simulink model "gm_inc_enc_v26_vnl"  (R2023a)
settings: Solver=FixedStepDiscrete  StartTime=0.0  StopTime=SimulationsDauer  RelTol=1e-3
undefined symbols (not defined in the file or in its folder): CW_CCW_Switch, d_axis_hit_CompareValue, DiscIntNeverNeededParam, f_ISR, IncPerTurn, inital_zero_speed_timeout, n_max, Offset_Position_elec, Offset_Position_mech, OmegaPerOverSampl, Periode, Phase_Delay_A, Phase_Delay_B, PolePair, QuadratureFactor, reciprocal_iterations, T_fpga, T_mech
libraries: simulink x25, hdlmdlgenlib x16, hdlsllib x4, dspsrcs4 x3, dspswit3 x2, spsEdgeDetectorLib x2, simulink_extras x1
(part 3 of 5)

== system gm_inc_enc_v26_vnl/IncEnc_V26_vnl/Check d-Axis-Hit ==
  Count_in : Inport
  IncPerTurn_elek_AXI4 : Inport  Port=2
  Constant : Constant  Value=0  OutDataTypeStr=Inherit: Inherit via back propagation  SampleTime=T_fpga
  Equal : RelationalOperator  Operator===  OutDataTypeStr=boolean  RndMeth=Simplest  InputSameDT=off
  Equal1 : RelationalOperator  Operator===  OutDataTypeStr=boolean  RndMeth=Simplest  InputSameDT=off
  OR : Logic  Operator=OR  AllPortsSameDT=off  OutDataTypeStr=boolean
  d-axis-hit : Outport  VectorParamsAs1DForOutWhenUnconnected=off
  wires:
  OR/1 -> d-axis-hit/1
  Equal1/1 -> OR/2
  Equal/1 -> OR/1
  IncPerTurn_elek_AXI4/1 -> Equal1/2
  Constant/1 -> Equal/2
  Count_in/1 -> Equal/1, Equal1/1

== system gm_inc_enc_v26_vnl/IncEnc_V26_vnl/Check d-Axis-Hit_WithCompare ==
  Count_in : Inport
  Counter_Compare : Inport  Port=2
  Equal : RelationalOperator  Operator===  OutDataTypeStr=boolean  RndMeth=Simplest  InputSameDT=off
  d-axis-hit : Outport  VectorParamsAs1DForOutWhenUnconnected=off
  wires:
  Equal/1 -> d-axis-hit/1
  Count_in/1 -> Equal/1
  Counter_Compare/1 -> Equal/2

== system gm_inc_enc_v26_vnl/IncEnc_V26_vnl/Counter ==
  note: Reset
  note: 1 for one cycle if edge recognized
  Enable_ctr : Inport
  I_line : Inport  Port=2
  Detec_edge : Sum  Inputs=+-  AccumDataTypeStr=int8  OutDataTypeStr=int8
  Reset_flag : Sum  Inputs=+-  AccumDataTypeStr=uint8  OutDataTypeStr=uint8
  reset_old : Delay  DelayLength=1
  reset_old1 : Delay  DelayLength=1
  reset_old_switch : Switch  Criteria=u2 ~= 0  SaturateOnIntegerOverflow=off  InputSameDT=off
  reset_old_switch1 : Switch  Criteria=u2 ~= 0  SaturateOnIntegerOverflow=off  InputSameDT=off
  Edge : Outport  VectorParamsAs1DForOutWhenUnconnected=off
  Reset : Outport  Port=2  VectorParamsAs1DForOutWhenUnconnected=off
  wires:
  Detec_edge/1 -> Edge/1, reset_old_switch1/2  "1 for one cycle if edge recognized"
  reset_old1/1 -> Detec_edge/2, reset_old_switch1/3
  reset_old_switch1/1 -> reset_old1/1
  Enable_ctr/1 -> reset_old_switch1/1, Detec_edge/1
  Reset_flag/1 -> reset_old_switch/2, Reset/1
  reset_old/1 -> Reset_flag/2, reset_old_switch/3
  reset_old_switch/1 -> reset_old/1
  I_line/1 -> reset_old_switch/1, Reset_flag/1

== system gm_inc_enc_v26_vnl/IncEnc_V26_vnl/Counter_Theta_el_wOffset ==
  note: Check if count is to small
  note: Count
  note: Check if count is to big 0-Increments
  Edge : Inport
  Reset : Inport  Port=2
  IncsPerTurn : Inport  Port=3
  Dir : Inport  Port=4
  Position_offset : Inport  Port=5
  Add1 : Sum  AccumDataTypeStr=int16  OutDataTypeStr=int16
  Constant1 : Constant  Value=0  OutDataTypeStr=int16  SampleTime=-1
  Constant2 : Constant  OutDataTypeStr=int16  SampleTime=-1
  Constant3 : Constant  Value=0  OutDataTypeStr=int16  SampleTime=-1
  Constant5 : Constant  Value=-1  OutDataTypeStr=int16  SampleTime=-1
  Relational Operator : RelationalOperator  Operator=>  OutDataTypeStr=boolean  InputSameDT=off
  Relational Operator1 : RelationalOperator  Operator=<=  OutDataTypeStr=boolean  InputSameDT=off
  Resett_switch1 : Switch  Criteria=u2 ~= 0  OutDataTypeStr=uint16  SaturateOnIntegerOverflow=off  InputSameDT=off
  Resett_switch2 : Switch  Criteria=u2 ~= 0  OutDataTypeStr=int16  SaturateOnIntegerOverflow=off  InputSameDT=off
  Resett_switch3 : Switch  Criteria=u2 ~= 0  OutDataTypeStr=int16  SaturateOnIntegerOverflow=off  InputSameDT=off
  Subsystem : Subsystem  Commented=on
  only_use_for_neg_speed : Switch  Threshold=1  SaturateOnIntegerOverflow=off  InputSameDT=off
  reset_old{1..7} (7 alike) : Delay  DelayLength=1
  speed_old_switch1 : Switch  Criteria=u2 ~= 0  SaturateOnIntegerOverflow=off  InputSameDT=off
  speed_old_switch2 : Switch  Threshold=1  SaturateOnIntegerOverflow=off  InputSameDT=off
  count : Outport  VectorParamsAs1DForOutWhenUnconnected=off
  wires:
  speed_old_switch1/1 -> Add1/1
  Constant5/1 -> speed_old_switch2/3
  Relational Operator/1 -> reset_old3/1
  Constant2/1 -> speed_old_switch2/1
  reset_old4/1 -> speed_old_switch1/1
  reset_old5/1 -> Resett_switch3/1, Relational Operator/2
  Resett_switch2/1 -> Resett_switch3/3
  only_use_for_neg_speed/1 -> Resett_switch3/2
  Resett_switch3/1 -> Relational Operator1/1, Resett_switch1/3
  speed_old_switch2/1 -> reset_old4/1
  Relational Operator1/1 -> reset_old2/1
  reset_old3/1 -> Resett_switch1/2
  Resett_switch1/1 -> Relational Operator/1, count/1, reset_old1/1
  Constant1/1 -> only_use_for_neg_speed/1, Relational Operator1/2, Resett_switch1/1
  Constant3/1 -> speed_old_switch1/3
  IncsPerTurn/1 -> reset_old5/1
  Reset/1 -> Resett_switch2/2
  reset_old2/1 -> only_use_for_neg_speed/3
  Edge/1 -> speed_old_switch1/2
  reset_old1/1 -> Add1/2
  Position_offset/1 -> reset_old7/1
  Add1/1 -> Resett_switch2/3
  Dir/1 -> reset_old6/1
  reset_old6/1 -> only_use_for_neg_speed/2, speed_old_switch2/2
  reset_old7/1 -> Resett_switch2/1

== system gm_inc_enc_v26_vnl/IncEnc_V26_vnl/Counter_position ==
  note: Check if count is to small
  note: Check if count is to big 0-Increments
  note: Count
  Edge : Inport
  Reset : Inport  Port=2
  IncsPerTurn : Inport  Port=3
  Dir : Inport  Port=4
  Add1 : Sum  AccumDataTypeStr=int16  OutDataTypeStr=int16
  Constant1 : Constant  Value=0  OutDataTypeStr=int16  SampleTime=-1
  Constant2 : Constant  OutDataTypeStr=int16  SampleTime=-1
  Constant3 : Constant  Value=0  OutDataTypeStr=int16  SampleTime=-1
  Constant4 : Constant  Value=0  OutDataTypeStr=int16  SampleTime=-1
  Constant5 : Constant  Value=-1  OutDataTypeStr=int16  SampleTime=-1
  Relational Operator : RelationalOperator  Operator=>  OutDataTypeStr=boolean  InputSameDT=off
  Relational Operator1 : RelationalOperator  Operator=<=  OutDataTypeStr=boolean  InputSameDT=off
  Resett_switch1 : Switch  Criteria=u2 ~= 0  OutDataTypeStr=uint16  SaturateOnIntegerOverflow=off  InputSameDT=off
  Resett_switch2 : Switch  Criteria=u2 ~= 0  OutDataTypeStr=int16  SaturateOnIntegerOverflow=off  InputSameDT=off
  Resett_switch3 : Switch  Criteria=u2 ~= 0  OutDataTypeStr=int16  SaturateOnIntegerOverflow=off  InputSameDT=off
  only_use_for_neg_speed : Switch  Threshold=1  SaturateOnIntegerOverflow=off  InputSameDT=off
  reset_old{1..6} (6 alike) : Delay  DelayLength=1
  speed_old_switch1 : Switch  Criteria=u2 ~= 0  SaturateOnIntegerOverflow=off  InputSameDT=off
  speed_old_switch2 : Switch  Threshold=1  SaturateOnIntegerOverflow=off  InputSameDT=off
  count : Outport  VectorParamsAs1DForOutWhenUnconnected=off
  wires:
  Constant1/1 -> Resett_switch2/1
  reset_old1/1 -> Add1/2
  reset_old5/1 -> Resett_switch3/1, Relational Operator/2
  reset_old2/1 -> only_use_for_neg_speed/3
  reset_old3/1 -> Resett_switch1/2
  Resett_switch1/1 -> count/1, reset_old1/1, Relational Operator/1
  reset_old6/1 -> speed_old_switch2/2, only_use_for_neg_speed/2
  IncsPerTurn/1 -> reset_old5/1
  reset_old4/1 -> speed_old_switch1/1
  only_use_for_neg_speed/1 -> Resett_switch3/2
  Relational Operator1/1 -> reset_old2/1
  Resett_switch3/1 -> Resett_switch1/3, Relational Operator1/1
  Resett_switch2/1 -> Resett_switch3/3
  Constant4/1 -> Resett_switch1/1, Relational Operator1/2, only_use_for_neg_speed/1
  Relational Operator/1 -> reset_old3/1
  speed_old_switch2/1 -> reset_old4/1
  Constant5/1 -> speed_old_switch2/3
  Dir/1 -> reset_old6/1
  Constant2/1 -> speed_old_switch2/1
  Constant3/1 -> speed_old_switch1/3
  speed_old_switch1/1 -> Add1/1
  Add1/1 -> Resett_switch2/3
  Edge/1 -> speed_old_switch1/2  "1 for one cycle if edge recognized"
  Reset/1 -> Resett_switch2/2

== system gm_inc_enc_v26_vnl/IncEnc_V26_vnl/Counter_position_wOffset ==
  note: Check if count is to big 0-Increments
  note: Count
  note: Check if count is to small
  Edge : Inport
  Reset : Inport  Port=2
  IncsPerTurn : Inport  Port=3
  Dir : Inport  Port=4
  Position_offset : Inport  Port=5
  Add1 : Sum  AccumDataTypeStr=int16  OutDataTypeStr=int16
  Constant1 : Constant  Value=0  OutDataTypeStr=int16  SampleTime=-1
  Constant2 : Constant  OutDataTypeStr=int16  SampleTime=-1
  Constant3 : Constant  Value=0  OutDataTypeStr=int16  SampleTime=-1
  Constant5 : Constant  Value=-1  OutDataTypeStr=int16  SampleTime=-1
  Relational Operator : RelationalOperator  Operator=>  OutDataTypeStr=boolean  InputSameDT=off
  Relational Operator1 : RelationalOperator  Operator=<=  OutDataTypeStr=boolean  InputSameDT=off
  Resett_switch1 : Switch  Criteria=u2 ~= 0  OutDataTypeStr=uint16  SaturateOnIntegerOverflow=off  InputSameDT=off
  Resett_switch2 : Switch  Criteria=u2 ~= 0  OutDataTypeStr=int16  SaturateOnIntegerOverflow=off  InputSameDT=off
  Resett_switch3 : Switch  Criteria=u2 ~= 0  OutDataTypeStr=int16  SaturateOnIntegerOverflow=off  InputSameDT=off
  Subsystem : Subsystem  Commented=on
  only_use_for_neg_speed : Switch  Threshold=1  SaturateOnIntegerOverflow=off  InputSameDT=off
  reset_old{1..7} (7 alike) : Delay  DelayLength=1
  speed_old_switch1 : Switch  Criteria=u2 ~= 0  SaturateOnIntegerOverflow=off  InputSameDT=off
  speed_old_switch2 : Switch  Threshold=1  SaturateOnIntegerOverflow=off  InputSameDT=off
  count : Outport  VectorParamsAs1DForOutWhenUnconnected=off
  wires:
  reset_old7/1 -> Resett_switch2/1
  reset_old6/1 -> speed_old_switch2/2, only_use_for_neg_speed/2
  Dir/1 -> reset_old6/1
  Add1/1 -> Resett_switch2/3
  Position_offset/1 -> reset_old7/1
  reset_old1/1 -> Add1/2
  Edge/1 -> speed_old_switch1/2
  reset_old2/1 -> only_use_for_neg_speed/3
  Reset/1 -> Resett_switch2/2
  IncsPerTurn/1 -> reset_old5/1
  Constant3/1 -> speed_old_switch1/3
  Constant1/1 -> Resett_switch1/1, Relational Operator1/2, only_use_for_neg_speed/1
  Resett_switch1/1 -> reset_old1/1, count/1, Relational Operator/1
  reset_old3/1 -> Resett_switch1/2
  Relational Operator1/1 -> reset_old2/1
  speed_old_switch2/1 -> reset_old4/1
  Resett_switch3/1 -> Resett_switch1/3, Relational Operator1/1
  only_use_for_neg_speed/1 -> Resett_switch3/2
  Resett_switch2/1 -> Resett_switch3/3
  reset_old5/1 -> Relational Operator/2, Resett_switch3/1
  reset_old4/1 -> speed_old_switch1/1
  Constant2/1 -> speed_old_switch2/1
  Relational Operator/1 -> reset_old3/1
  Constant5/1 -> speed_old_switch2/3
  speed_old_switch1/1 -> Add1/1

== system gm_inc_enc_v26_vnl/IncEnc_V26_vnl/Direction ==
  A : Inport
  B : Inport  Port=2
  Add : Sum  Inputs=+-  AccumDataTypeStr=fixdt(1,4,0)  OutDataTypeStr=fixdt(1,4,0)
  Add1 : Sum  Inputs=+-  AccumDataTypeStr=fixdt(1,4,0)  OutDataTypeStr=fixdt(1,4,0)
  Add2 : Sum  AccumDataTypeStr=fixdt(1,4,0)  OutDataTypeStr=fixdt(1,4,0)
  Change : Sum  AccumDataTypeStr=fixdt(1,4,0)  OutDataTypeStr=fixdt(1,4,0)
  Change1 : Delay  DelayLength=1
  Save_Direction : Switch  Criteria=u2 ~= 0  Threshold=0.1  OutDataTypeStr=fixdt(1,4,0)  SaturateOnIntegerOverflow=off  InputSameDT=off
  T_count_switch : Switch  Threshold=1  OutDataTypeStr=Inherit: Inherit via back propagation  SaturateOnIntegerOverflow=off  InputSameDT=off
  TrnLeft : Sum  Inputs=+-  AccumDataTypeStr=fixdt(1,4,0)  OutDataTypeStr=fixdt(1,4,0)
  TrnRight : Sum  Inputs=+-  AccumDataTypeStr=fixdt(1,4,0)  OutDataTypeStr=fixdt(1,4,0)
  TurnLeft : Constant  Value=-1  OutDataTypeStr=fixdt(1,4,0)  SampleTime=-1
  TurnRight : Constant  OutDataTypeStr=fixdt(1,4,0)  SampleTime=-1
  count_old : Delay  DelayLength=1
  count_old1 : Delay  DelayLength=1
  count_old2 : Delay  DelayLength=1
  count_old_switch : Switch  Criteria=u2 ~= 0  OutDataTypeStr=Inherit: Inherit via back propagation  SaturateOnIntegerOverflow=off  InputSameDT=off
  count_old_switch1 : Switch  Criteria=u2 ~= 0  OutDataTypeStr=Inherit: Inherit via back propagation  SaturateOnIntegerOverflow=off  InputSameDT=off
  new_value : Delay  DelayLength=1
  nothing : Constant  Value=0  OutDataTypeStr=fixdt(1,4,0)  SampleTime=-1
  nothing1 : Constant  Value=0  OutDataTypeStr=fixdt(1,4,0)  SampleTime=-1
  speed_old_switch : Switch  Threshold=1  OutDataTypeStr=Inherit: Inherit via back propagation  SaturateOnIntegerOverflow=off  InputSameDT=off
  Dir : Outport  VectorParamsAs1DForOutWhenUnconnected=off
  wires:
  count_old2/1 -> Dir/1, Save_Direction/3  "Dir"
  Change1/1 -> Save_Direction/2  "Change"
  Change/1 -> Change1/1
  Add2/1 -> new_value/1
  speed_old_switch/1 -> Add2/2, Change/2
  nothing1/1 -> T_count_switch/3
  nothing/1 -> speed_old_switch/3
  TurnLeft/1 -> speed_old_switch/1
  TrnLeft/1 -> speed_old_switch/2  "TrnLeft"
  new_value/1 -> Save_Direction/1
  TrnRight/1 -> T_count_switch/2  "Trn_Right"
  Add1/1 -> count_old_switch1/2, TrnLeft/1  "Edge_B"
  count_old1/1 -> Add1/2, count_old_switch1/3
  count_old_switch1/1 -> count_old1/1
  B/1 -> count_old_switch1/1, Add1/1, TrnRight/2
  Save_Direction/1 -> count_old2/1
  T_count_switch/1 -> Add2/1, Change/1
  Add/1 -> count_old_switch/2, TrnRight/1  "Edge_A"
  TurnRight/1 -> T_count_switch/1
  count_old/1 -> Add/2, count_old_switch/3
  count_old_switch/1 -> count_old/1
  A/1 -> count_old_switch/1, Add/1, TrnLeft/2

== system gm_inc_enc_v26_vnl/IncEnc_V26_vnl/Index_Latch ==
  Reset_in : Inport
  Constant : Constant  OutDataTypeStr=boolean  SampleTime=T_fpga
  Constant4 : Constant  Value=0  OutDataTypeStr=boolean  SampleTime=T_fpga
  Delay : Delay  DelayLength=1
  OR : Logic  Operator=OR  AllPortsSameDT=off  OutDataTypeStr=boolean
  Switch : Switch  Criteria=u2 > Threshold  SaturateOnIntegerOverflow=off  InputSameDT=off
  Index_found : Outport
  wires:
  OR/1 -> Switch/2
  Reset_in/1 -> OR/1
  Switch/1 -> Delay/1, Index_found/1
  Constant/1 -> Switch/1
  Delay/1 -> OR/2
  Constant4/1 -> Switch/3

== system gm_inc_enc_v26_vnl/IncEnc_V26_vnl/count_lines ==
  note: omega by counting lines, can be used for high-speed, but is not recommended for small drives!
      | However, for using this approach, we need a quite long time window in order to get an accurate speed.
      | For small drives a long time window is not acceptable, since the mechanical time constant is small.
      | e.g. using just 100us (since the speed control has this period at 10kHz) we can calculate as following:
      | speed = 5034rpm, Increments = 5000, QuadratureFactor = 4, f_cc = 10000 kHz
      | In the test, 169 lines are counted in 100us in the described example.
      | -> 169*(10000/(4*5000))*60 = 5070rpm (so this is not accurate!)
      | However, a longer time window is not acceptabel for speed control with10kHz. More increments is not common, since 5000 are already a lot!
  note: Count
  note: Check if count is to big in order to safe for value overflow
  note: Set new counter value
  Edge : Inport
  Reset : Inport  Port=2
  IncsPerTurn : Inport  Port=3
  Add1 : Sum  AccumDataTypeStr=int16  OutDataTypeStr=int16
  Constant1 : Constant  Value=0  OutDataTypeStr=int16  SampleTime=-1
  Constant2 : Constant  OutDataTypeStr=int16  SampleTime=-1
  Constant3 : Constant  Value=0  OutDataTypeStr=int16  SampleTime=-1
  Constant4 : Constant  Value=10  OutDataTypeStr=int16  SampleTime=-1
  Relational Operator : RelationalOperator  Operator=>  OutDataTypeStr=boolean  InputSameDT=off
  Reset_when_overflow : Sum  OutDataTypeStr=int16
  Resett_switch1 : Switch  Criteria=u2 ~= 0  OutDataTypeStr=int16  SaturateOnIntegerOverflow=off  InputSameDT=off
  Resett_switch2 : Switch  Criteria=u2 ~= 0  OutDataTypeStr=int16  SaturateOnIntegerOverflow=off  InputSameDT=off
  reset_old{1,3..5} (4 alike) : Delay  DelayLength=1
  reset_old_switch1 : Switch  Criteria=u2 ~= 0  SaturateOnIntegerOverflow=off  InputSameDT=off
  speed_old_switch1 : Switch  Criteria=u2 ~= 0  SaturateOnIntegerOverflow=off  InputSameDT=off
  count : Outport  VectorParamsAs1DForOutWhenUnconnected=off
  wires:
  reset_old_switch1/1 -> count/1, reset_old1/1
  Reset/1 -> Resett_switch2/2, reset_old_switch1/2  "Use new value"
  reset_old1/1 -> reset_old_switch1/3
  reset_old3/1 -> Relational Operator/1, Add1/2, reset_old_switch1/1
  Resett_switch1/1 -> reset_old3/1
  Constant4/1 -> Reset_when_overflow/1
  Constant2/1 -> reset_old4/1
  Add1/1 -> Resett_switch2/3
  IncsPerTurn/1 -> Reset_when_overflow/2
  Constant3/1 -> speed_old_switch1/3
  Constant1/1 -> Resett_switch1/1, Resett_switch2/1
  Edge/1 -> speed_old_switch1/2  "1 for one cycle if edge recognized"
  reset_old4/1 -> speed_old_switch1/1
  Resett_switch2/1 -> Resett_switch1/3
  reset_old5/1 -> Relational Operator/2
  speed_old_switch1/1 -> Add1/1
  Relational Operator/1 -> Resett_switch1/2
  Reset_when_overflow/1 -> reset_old5/1

== system gm_inc_enc_v26_vnl/IncEnc_V26_vnl/digital_filter ==
  A : Inport
  AND : Logic  Inputs=3  IconShape=distinctive  AllPortsSameDT=off  OutDataTypeStr=boolean
  AND1 : Logic  Inputs=3  IconShape=distinctive  AllPortsSameDT=off  OutDataTypeStr=boolean
  Delay1 : Delay  DelayLength=1
  Delay2 : Delay  DelayLength=1
  Delay3 : Delay  DelayLength=1
  NOT : Logic  Operator=NOT  IconShape=distinctive  AllPortsSameDT=off  OutDataTypeStr=boolean
  NOT1 : Logic  Operator=NOT  IconShape=distinctive  AllPortsSameDT=off  OutDataTypeStr=boolean
  NOT2 : Logic  Operator=NOT  IconShape=distinctive  AllPortsSameDT=off  OutDataTypeStr=boolean
  Subsystem1 : Subsystem
  Q : Outport
  wires:
  AND/1 -> Subsystem1/1(S)
  AND1/1 -> Subsystem1/2(R)
  Subsystem1/1(Q) -> Q/1
  Delay1/1 -> Delay2/1, NOT/1, AND/1
  Delay2/1 -> Delay3/1, NOT1/1, AND/2
  Delay3/1 -> NOT2/1, AND/3
  NOT/1 -> AND1/1
  NOT1/1 -> AND1/2
  NOT2/1 -> AND1/3
  A/1 -> Delay1/1

== system gm_inc_enc_v26_vnl/IncEnc_V26_vnl/digital_filter1 ==
  A : Inport
  AND : Logic  Inputs=3  IconShape=distinctive  AllPortsSameDT=off  OutDataTypeStr=boolean
  AND1 : Logic  Inputs=3  IconShape=distinctive  AllPortsSameDT=off  OutDataTypeStr=boolean
  Delay1 : Delay  DelayLength=1
  Delay2 : Delay  DelayLength=1
  Delay3 : Delay  DelayLength=1
  NOT : Logic  Operator=NOT  IconShape=distinctive  AllPortsSameDT=off  OutDataTypeStr=boolean
  NOT1 : Logic  Operator=NOT  IconShape=distinctive  AllPortsSameDT=off  OutDataTypeStr=boolean
  NOT2 : Logic  Operator=NOT  IconShape=distinctive  AllPortsSameDT=off  OutDataTypeStr=boolean
  Subsystem1 : Subsystem
  Q : Outport
  wires:
  A/1 -> Delay1/1
  NOT2/1 -> AND1/3
  NOT1/1 -> AND1/2
  NOT/1 -> AND1/1
  Delay3/1 -> AND/3, NOT2/1
  Delay2/1 -> AND/2, NOT1/1, Delay3/1
  Delay1/1 -> AND/1, NOT/1, Delay2/1
  Subsystem1/1(Q) -> Q/1
  AND1/1 -> Subsystem1/2(R)
  AND/1 -> Subsystem1/1(S)

== system gm_inc_enc_v26_vnl/IncEnc_V26_vnl/digital_filter2 ==
  A : Inport
  AND : Logic  Inputs=3  IconShape=distinctive  AllPortsSameDT=off  OutDataTypeStr=boolean
  AND1 : Logic  Inputs=3  IconShape=distinctive  AllPortsSameDT=off  OutDataTypeStr=boolean
  Delay1 : Delay  DelayLength=1
  Delay2 : Delay  DelayLength=1
  Delay3 : Delay  DelayLength=1
  NOT : Logic  Operator=NOT  IconShape=distinctive  AllPortsSameDT=off  OutDataTypeStr=boolean
  NOT1 : Logic  Operator=NOT  IconShape=distinctive  AllPortsSameDT=off  OutDataTypeStr=boolean
  NOT2 : Logic  Operator=NOT  IconShape=distinctive  AllPortsSameDT=off  OutDataTypeStr=boolean
  Subsystem1 : Subsystem
  Q : Outport
  wires:
  AND/1 -> Subsystem1/1(S)
  AND1/1 -> Subsystem1/2(R)
  Subsystem1/1(Q) -> Q/1
  Delay1/1 -> Delay2/1, NOT/1, AND/1
  Delay2/1 -> Delay3/1, NOT1/1, AND/2
  Delay3/1 -> NOT2/1, AND/3
  NOT/1 -> AND1/1
  NOT1/1 -> AND1/2
  NOT2/1 -> AND1/3
  A/1 -> Delay1/1

== system gm_inc_enc_v26_vnl/IncEnc_V26_vnl/speed1 ==
  A : Inport
  B : Inport  Port=2
  Dir : Inport  Port=3
  OmegaPerOverSampl : Inport  Port=4
  T : Inport  Port=5
  timeout_value : Inport  Port=6  OutDataTypeStr=uint32
  Average : Subsystem
  Delay{1..3,6} (4 alike) : Delay  DelayLength=1  InitialCondition=0
  Demux : Demux
  Logical1 : Logic  Operator=NOT  AllPortsSameDT=off  OutDataTypeStr=boolean
  Logical2 : Logic  Operator=NOT  AllPortsSameDT=off  OutDataTypeStr=boolean
  Mux : Mux
  OR1 : Logic  Operator=OR  Inputs=1  AllPortsSameDT=off  OutDataTypeStr=boolean
  OR2 : Logic  Operator=OR  Inputs=1  AllPortsSameDT=off  OutDataTypeStr=boolean
  OS_factor_logic : Subsystem
      settings: PortSchema="{\"entries\":[{\"content\":{\"sides\":[{\"content\":{\"connectorIds\":[\"In1\",\"In2\",\"In3\",\"In4\",\"Out2\"]},\"type\":\"ConnectorPlacement.EquallySpacedRectSide\",\"uuid\":\"00190a63-1990-4dc8-8561-af6346041cd2\"},{\"content\":{\"connectorIds\":[\"Out1\",\"In5\"],\"side\":\"RIGHT\"},\"type\":\"ConnectorPlacement.EquallySpacedRectSide\",\"uuid\":\"ed8fa1bb-ba76-4f60-9676-d72d7f094a86\"},{\"content\":{\"connectorIds\":[],\"side\":\"TOP\"},\"type\":\"ConnectorPlacement.EquallySpacedRectSide\",\"uuid\":\"16aa4cab-6298-4523-a92b-d078d21511a0\"}]},\"type\":\"ConnectorPlacement.EquallySpacedConnector\",\"uuid\":\"bb0c721d-662f-49b4-b1e3-cc7ff0334cdb\"}],\"packageUris\":[\"http://schema.mathworks.com/mf0/Connector/R2020b\"],\"version\":\"1.0\"}"
  calc_omega : Subsystem  TreatAsAtomicUnit=on
  omega : Outport  VectorParamsAs1DForOutWhenUnconnected=off
  OverSamplFactor : Outport  Port=2
  omega_MA_N4 : Outport  Port=3  VectorParamsAs1DForOutWhenUnconnected=off
  timeout_active : Outport  Port=4  OutDataTypeStr=boolean  VectorParamsAs1DForOutWhenUnconnected=off
  omegaA : Outport  Port=5  VectorParamsAs1DForOutWhenUnconnected=off
  omegaB : Outport  Port=6  VectorParamsAs1DForOutWhenUnconnected=off
  omegaNOTA : Outport  Port=7  VectorParamsAs1DForOutWhenUnconnected=off
  omegaNOTB : Outport  Port=8  VectorParamsAs1DForOutWhenUnconnected=off
  new_measurement : Outport  Port=9  OutDataTypeStr=boolean  VectorParamsAs1DForOutWhenUnconnected=off
  wires:
  Average/1(Omega) -> omega/1
  Delay3/1 -> Mux/4
  Delay2/1 -> Mux/3
  Delay1/1 -> Mux/2
  Delay6/1 -> Mux/1
  OS_factor_logic/1(oversampling_adjusted) -> calc_omega/4(oversampling_state)
  Logical1/1 -> Delay3/1  "NOT_B"
  Logical2/1 -> Delay2/1  "NOT_A"
  calc_omega/4(timeout_active) -> OR1/1
  calc_omega/3(state_count_edges) -> OS_factor_logic/3(state_edges)
  calc_omega/2(NewMeasurement) -> OS_factor_logic/1(new_transisiton), OR2/1  "newMeas"
  calc_omega/1(omega_oversampled) -> Average/1("OmegaIn "), Demux/1  "omega"
  Demux/3 -> omegaNOTA/1
  Demux/4 -> omegaNOTB/1
  Demux/1 -> omegaA/1
  Demux/2 -> omegaB/1
  timeout_value/1 -> calc_omega/5(timeout_value)
  T/1 -> calc_omega/3(T)
  Mux/1 -> calc_omega/1(Encoder Line)
  A/1 -> Delay6/1, Logical2/1  "A"
  Average/2(OmegaOut_MA_N4) -> OS_factor_logic/4(omega), omega_MA_N4/1  "final omega oversampled"
  OR1/1 -> timeout_active/1  "timeout_active_all_ORed"
  OS_factor_logic/2(oversampling_state) -> OverSamplFactor/1  "OS_B"
  OR2/1 -> new_measurement/1, Average/2(NewMeasurement), OS_factor_logic/2(Allow_ToCheckOversampling)  "newMeas_allORed"
  OmegaPerOverSampl/1 -> OS_factor_logic/5(OverSamplOmega)
  B/1 -> Logical1/1, Delay1/1  "B"
  Dir/1 -> calc_omega/2(Dir)

== system gm_inc_enc_v26_vnl/Testfield/Counter_position_wOffset ==
  note: Check if count is to small
  note: Count
  note: Check if count is to big 0-Increments
  Edge : Inport
  Reset : Inport  Port=2
  IncsPerTurn : Inport  Port=3
  Dir : Inport  Port=4
  Position_offset : Inport  Port=5
  Add1 : Sum  AccumDataTypeStr=int16  OutDataTypeStr=int16
  Constant1 : Constant  Value=0  OutDataTypeStr=int16  SampleTime=-1
  Constant2 : Constant  OutDataTypeStr=int16  SampleTime=-1
  Constant3 : Constant  Value=0  OutDataTypeStr=int16  SampleTime=-1
  Constant5 : Constant  Value=-1  OutDataTypeStr=int16  SampleTime=-1
  Relational Operator : RelationalOperator  Operator=>  OutDataTypeStr=boolean  InputSameDT=off
  Relational Operator1 : RelationalOperator  Operator=<=  OutDataTypeStr=boolean  InputSameDT=off
  Resett_switch1 : Switch  Criteria=u2 ~= 0  OutDataTypeStr=uint16  SaturateOnIntegerOverflow=off  InputSameDT=off
  Resett_switch2 : Switch  Criteria=u2 ~= 0  OutDataTypeStr=int16  SaturateOnIntegerOverflow=off  InputSameDT=off
  Resett_switch3 : Switch  Criteria=u2 ~= 0  OutDataTypeStr=int16  SaturateOnIntegerOverflow=off  InputSameDT=off
  Subsystem : Subsystem  Commented=on
  only_use_for_neg_speed : Switch  Threshold=1  SaturateOnIntegerOverflow=off  InputSameDT=off
  reset_old{1..7} (7 alike) : Delay  DelayLength=1
  speed_old_switch1 : Switch  Criteria=u2 ~= 0  SaturateOnIntegerOverflow=off  InputSameDT=off
  speed_old_switch2 : Switch  Threshold=1  SaturateOnIntegerOverflow=off  InputSameDT=off
  count : Outport  VectorParamsAs1DForOutWhenUnconnected=off
  wires:
  speed_old_switch1/1 -> Add1/1
  Constant5/1 -> speed_old_switch2/3
  Relational Operator/1 -> reset_old3/1
  Constant2/1 -> speed_old_switch2/1
  reset_old4/1 -> speed_old_switch1/1
  reset_old5/1 -> Resett_switch3/1, Relational Operator/2
  Resett_switch2/1 -> Resett_switch3/3
  only_use_for_neg_speed/1 -> Resett_switch3/2
  Resett_switch3/1 -> Relational Operator1/1, Resett_switch1/3
  speed_old_switch2/1 -> reset_old4/1
  Relational Operator1/1 -> reset_old2/1
  reset_old3/1 -> Resett_switch1/2
  Resett_switch1/1 -> Relational Operator/1, count/1, reset_old1/1
  Constant1/1 -> only_use_for_neg_speed/1, Relational Operator1/2, Resett_switch1/1
  Constant3/1 -> speed_old_switch1/3
  IncsPerTurn/1 -> reset_old5/1
  Reset/1 -> Resett_switch2/2
  reset_old2/1 -> only_use_for_neg_speed/3
  Edge/1 -> speed_old_switch1/2
  reset_old1/1 -> Add1/2
  Position_offset/1 -> reset_old7/1
  Add1/1 -> Resett_switch2/3
  Dir/1 -> reset_old6/1
  reset_old6/1 -> only_use_for_neg_speed/2, speed_old_switch2/2
  reset_old7/1 -> Resett_switch2/1

== system gm_inc_enc_v26_vnl/Testfield/Index_Latch ==
  Reset_in : Inport
  Constant : Constant  OutDataTypeStr=boolean
  Constant4 : Constant  Value=0  OutDataTypeStr=boolean
  Delay : Delay  DelayLength=1
  OR : Logic  Operator=OR  AllPortsSameDT=off  OutDataTypeStr=boolean
  Switch : Switch  Criteria=u2 > Threshold  SaturateOnIntegerOverflow=off  InputSameDT=off
  Index_found : Outport
  wires:
  Constant4/1 -> Switch/3
  Delay/1 -> OR/2
  Constant/1 -> Switch/1
  Switch/1 -> Index_found/1, Delay/1
  Reset_in/1 -> OR/1
  OR/1 -> Switch/2

== system gm_inc_enc_v26_vnl/Create_Referenz/IncrementalEncoder_Floating/CutTheta_0_2PI ==
  In1 : Inport
  Add7 : Sum  Inputs=+-  OutDataTypeStr=double
  Gain : Gain  Gain=1/(2*pi)
  Gain11 : Gain  Gain=2*pi
  Rounding Function : Rounding
  Out1 : Outport  VectorParamsAs1DForOutWhenUnconnected=off
  wires:
  Gain/1 -> Rounding Function/1
  Rounding Function/1 -> Gain11/1
  Gain11/1 -> Add7/2
  In1/1 -> Gain/1, Add7/1
  Add7/1 -> Out1/1

== system gm_inc_enc_v26_vnl/Create_Referenz/IncrementalEncoder_Floating/n_aus_theta_v4 ==
  theta : Inport
  Abs : Abs  SaturateOnIntegerOverflow=off
  Add : Sum  Inputs=-+
  Add1 : Sum  Inputs=+-
  Gain : Gain  Gain=2*pi
  Gain1 : Gain  Gain=1/T_mech
  Gain2 : Gain  Gain=60/(2*pi)
  Geschwindigkeitsfilter1 : Subsystem
  Rate Limiter2 1/T : RateLimiter  RisingSlewLimit=1/T_mech*10  FallingSlewLimit=-1/T_mech*10  SampleTimeMode=inherited
  Saturation : Saturate  UpperLimit=n_max  LowerLimit=-n_max
  Scope1 : Scope  NumInputPorts=5
  Scope2 : Scope  NumInputPorts=5
  Sign : Signum
  Switch : Switch  Threshold=3  SaturateOnIntegerOverflow=off  InputSameDT=off
  Unit Delay : UnitDelay  SampleTime=-1  HasFrameUpgradeWarning=on
  n : Outport  VectorParamsAs1DForOutWhenUnconnected=off
  wires:
  Switch/1 -> Scope1/3, Gain1/1
  Add/1 -> Scope2/1, Switch/1
  Gain/1 -> Add/1
  Sign/1 -> Gain/1
  Add1/1 -> Scope2/3, Add/2, Abs/1, Scope2/2, Switch/3, Sign/1
  Abs/1 -> Scope1/4, Switch/2
  Gain1/1 -> Scope1/2, Gain2/1
  theta/1 -> Scope2/5, Add1/1, Unit Delay/1
  Unit Delay/1 -> Scope2/4, Add1/2
  Gain2/1 -> Saturation/1
  Geschwindigkeitsfilter1/1(Out1) -> Scope1/5, Rate Limiter2 1/T/1
  Rate Limiter2 1/T/1 -> n/1
  Saturation/1 -> Scope1/1, Geschwindigkeitsfilter1/1(In1)

== system gm_inc_enc_v26_vnl/IncEnc_V26/digital_filter/Subsystem1 ==
  S : Inport  OutDataTypeStr=boolean  PortDimensions=1  SampleTime=1e-08
  R : Inport  Port=2  OutDataTypeStr=boolean  PortDimensions=1  SampleTime=1e-08
  AND : Logic  Operator=NOR  AllPortsSameDT=off  OutDataTypeStr=boolean  SampleTime=1e-08
  AND1 : Logic  Operator=NOR  AllPortsSameDT=off  OutDataTypeStr=boolean  SampleTime=1e-08
  Delay : Delay  DelayLength=double(1)  InitialCondition=0  SampleTime=1e-08
  Q : Outport  SampleTime=1e-08
  wires:
  AND1/1 -> AND/2
  Delay/1 -> AND1/1
  AND/1 -> Delay/1, Q/1
  R/1 -> AND/1
  S/1 -> AND1/2

== system gm_inc_enc_v26_vnl/IncEnc_V26/digital_filter1/Subsystem1 ==
  S : Inport  OutDataTypeStr=boolean  PortDimensions=1  SampleTime=1e-08
  R : Inport  Port=2  OutDataTypeStr=boolean  PortDimensions=1  SampleTime=1e-08
  AND : Logic  Operator=NOR  AllPortsSameDT=off  OutDataTypeStr=boolean  SampleTime=1e-08
  AND1 : Logic  Operator=NOR  AllPortsSameDT=off  OutDataTypeStr=boolean  SampleTime=1e-08
  Delay : Delay  DelayLength=double(1)  InitialCondition=0  SampleTime=1e-08
  Q : Outport  SampleTime=1e-08
  wires:
  AND1/1 -> AND/2
  Delay/1 -> AND1/1
  AND/1 -> Delay/1, Q/1
  R/1 -> AND/1
  S/1 -> AND1/2

== system gm_inc_enc_v26_vnl/IncEnc_V26/digital_filter2/Subsystem1 ==
  S : Inport  OutDataTypeStr=boolean  PortDimensions=1  SampleTime=1e-08
  R : Inport  Port=2  OutDataTypeStr=boolean  PortDimensions=1  SampleTime=1e-08
  AND : Logic  Operator=NOR  AllPortsSameDT=off  OutDataTypeStr=boolean  SampleTime=1e-08
  AND1 : Logic  Operator=NOR  AllPortsSameDT=off  OutDataTypeStr=boolean  SampleTime=1e-08
  Delay : Delay  DelayLength=double(1)  InitialCondition=0  SampleTime=1e-08
  Q : Outport  SampleTime=1e-08
  wires:
  AND1/1 -> AND/2
  Delay/1 -> AND1/1
  AND/1 -> Delay/1, Q/1
  R/1 -> AND/1
  S/1 -> AND1/2

== system gm_inc_enc_v26_vnl/IncEnc_V26/speed1/Average ==
  note: average 4 parallel measurements
  note: moving average of 4 last measurements, which in total results in a moving average of the last 8 samples
  "OmegaIn " : Inport  OutDataTypeStr=fixdt(1, 24, 11)  PortDimensions=[4]  SampleTime=1e-08
  NewMeasurement : Inport  Port=2  OutDataTypeStr=boolean  PortDimensions=1  SampleTime=1e-08
  Delay_Switch : Switch  Criteria=u2 ~= 0  Threshold=double(0)  OutDataTypeStr=fixdt(1, 24, 11)  SampleTime=1e-08  SaturateOnIntegerOverflow=off  InputSameDT=off
  Delay_Switch1 : Switch  Criteria=u2 ~= 0  Threshold=double(0)  OutDataTypeStr=fixdt(1, 24, 11)  SampleTime=1e-08  SaturateOnIntegerOverflow=off  InputSameDT=off
  Delay_Switch2 : Switch  Criteria=u2 ~= 0  Threshold=double(0)  OutDataTypeStr=fixdt(1, 24, 11)  SampleTime=1e-08  SaturateOnIntegerOverflow=off  InputSameDT=off
  Gain : Gain  Gain="fi(0,1,26,26,\"hex\",\"1000000\")"  ParamDataTypeStr=fixdt(1, 26, 26)  OutDataTypeStr=fixdt(1, 24, 11)  SampleTime=1e-08
  Gain1 : Gain  Gain="fi(0,1,26,26,\"hex\",\"1000000\")"  ParamDataTypeStr=fixdt(1, 26, 26)  OutDataTypeStr=fixdt(1, 24, 11)  SampleTime=1e-08
  Sum of Elements{1..2,4..5} (4 alike) : Sum  AccumDataTypeStr=fixdt(1, 25, 11)  OutDataTypeStr=fixdt(1, 25, 11)  SampleTime=1e-08
  Sum of Elements3 : Sum  AccumDataTypeStr=fixdt(1, 26, 11)  OutDataTypeStr=fixdt(1, 26, 11)  SampleTime=1e-08
  Sum of Elements6 : Sum  AccumDataTypeStr=fixdt(1, 26, 11)  OutDataTypeStr=fixdt(1, 26, 11)  SampleTime=1e-08
  rd_{0..8} (9 alike) : Delay  DelayLength=double(1)  InitialCondition=0  SampleTime=1e-08
  t : Demux
  t{1..6} (6 alike) : hdlmdlgenlib/Buffer
  Omega : Outport  SampleTime=1e-08  VectorParamsAs1DForOutWhenUnconnected=off
  OmegaOut_MA_N4 : Outport  Port=2  SampleTime=1e-08  VectorParamsAs1DForOutWhenUnconnected=off
  wires:
  rd_5/1 -> Delay_Switch2/2, Delay_Switch1/2, Delay_Switch/2
  t2/1 -> rd_5/1
  rd_8/1 -> Sum of Elements2/2, Delay_Switch2/3
  t6/1 -> rd_8/1
  rd_7/1 -> Sum of Elements2/1, Delay_Switch2/1, Delay_Switch1/3
  t5/1 -> rd_7/1
  rd_6/1 -> Sum of Elements1/2, Delay_Switch/3, Delay_Switch1/1
  t4/1 -> rd_6/1
  rd_4/1 -> Sum of Elements1/1
  rd_1/1 -> Sum of Elements5/1
  rd_3/1 -> Sum of Elements5/2
  rd_2/1 -> Sum of Elements4/2
  rd_0/1 -> Sum of Elements4/1
  Delay_Switch2/1 -> t6/1
  Delay_Switch1/1 -> t5/1
  Delay_Switch/1 -> t4/1
  NewMeasurement/1 -> t2/1
  "OmegaIn "/1 -> t/1
  t/4 -> rd_3/1
  t/3 -> rd_1/1
  t/2 -> rd_2/1
  t/1 -> rd_0/1
  t3/1 -> rd_4/1
  Sum of Elements6/1 -> Gain1/1
  Sum of Elements5/1 -> Sum of Elements6/2
  Sum of Elements4/1 -> Sum of Elements6/1
  Sum of Elements3/1 -> Gain/1
  Sum of Elements2/1 -> Sum of Elements3/2
  Sum of Elements1/1 -> Sum of Elements3/1
  Gain1/1 -> t1/1
  Gain/1 -> OmegaOut_MA_N4/1
  t1/1 -> Delay_Switch/1, Omega/1, t3/1

== system gm_inc_enc_v26_vnl/IncEnc_V26/speed1/OS_factor_logic ==
  new_transisiton : Inport  OutDataTypeStr=boolean  PortDimensions=[4]  SampleTime=1e-08
  Allow_ToCheckOversampling : Inport  Port=2  OutDataTypeStr=boolean  PortDimensions=1  SampleTime=1e-08
  state_edges : Inport  Port=3  OutDataTypeStr=int16  PortDimensions=[4]  SampleTime=1e-08
  omega : Inport  Port=4  OutDataTypeStr=fixdt(1, 24, 11)  PortDimensions=1  SampleTime=1e-08
  OverSamplOmega : Inport  Port=5  OutDataTypeStr=fixdt(1, 24, 11)  PortDimensions=1  SampleTime=1e-08
  Abs : Abs  SampleTime=1e-08  OutDataTypeStr=fixdt(1, 24, 11)  SaturateOnIntegerOverflow=off
  Data Type Conversion1 : DataTypeConversion  OutDataTypeStr=fixdt(0,16,0)
  Delay7_Initial_Val : Constant  OutDataTypeStr=uint16  SampleTime=1e-08
  Delay7_ctrl_const : Constant  OutDataTypeStr=boolean  SampleTime=1e-08
  Delay7_switch : Switch  Criteria=u2 ~= 0  Threshold=double(0)  OutDataTypeStr=uint16  SampleTime=1e-08  SaturateOnIntegerOverflow=off  InputSameDT=off
  Sum : Sum  Inputs=+-  AccumDataTypeStr=uint16  OutDataTypeStr=uint16  SampleTime=1e-08
  align_oversamples : Subsystem
  oversample_factor : Subsystem
  rd_{0..3} (4 alike) : Delay  DelayLength=double(1)  InitialCondition=0  SampleTime=1e-08
  oversampling_adjusted : Outport  PortDimensions=4  SampleTime=1e-08
  oversampling_state : Outport  Port=2  SampleTime=1e-08
  wires:
  rd_0/1 -> Delay7_switch/2
  rd_1/1 -> oversample_factor/5(InternalOmega)
  rd_2/1 -> Delay7_switch/1
  rd_3/1 -> Sum/2
  Delay7_ctrl_const/1 -> rd_0/1
  Delay7_Initial_Val/1 -> Delay7_switch/3
  oversample_factor/2(InternalOmega_Out) -> rd_1/1
  oversample_factor/1(state_Out) -> rd_2/1
  align_oversamples/1(delay_output) -> rd_3/1
  Sum/1 -> oversampling_adjusted/1
  Delay7_switch/1 -> align_oversamples/1(oversampling_factor), oversample_factor/4(state), Data Type Conversion1/1, Sum/1
  Data Type Conversion1/1 -> oversampling_state/1
  Abs/1 -> oversample_factor/2(ReadBack_Omega)
  OverSamplOmega/1 -> oversample_factor/3(OverSamplOmega)
  omega/1 -> Abs/1
  state_edges/1 -> align_oversamples/3(states)
  Allow_ToCheckOversampling/1 -> oversample_factor/1(AllowCheckOverSampl)
  new_transisiton/1 -> align_oversamples/2(new_transition)

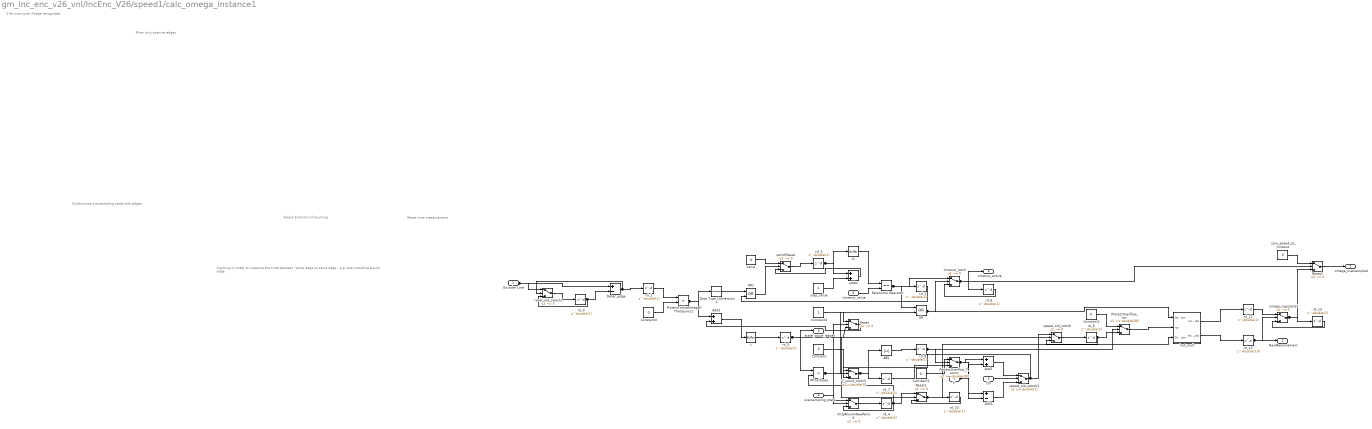
== system gm_inc_enc_v26_vnl/IncEnc_V26/speed1/calc_omega_instance1 ==
  note: Synchronize oversampling state with edges
  note: Filter only positive edges
  note: Select direction of counting
  note: 1 for one cycle if edge recognized
  note: Reset time measurement
  note: Count up in order to measure the time between "same edge to same edge", e.g. every positive A-Line edge
  Encoder Line : Inport  OutDataTypeStr=boolean  PortDimensions=1  SampleTime=1e-08
  Dir : Inport  Port=2  OutDataTypeStr=fixdt(1, 4, 0)  PortDimensions=1  SampleTime=1e-08
  T : Inport  Port=3  OutDataTypeStr=fixdt(1, 38, 32)  PortDimensions=1  SampleTime=1e-08
  oversampling_state : Inport  Port=4  OutDataTypeStr=uint16  PortDimensions=1  SampleTime=1e-08
  timeout_value : Inport  Port=5  OutDataTypeStr=uint32  PortDimensions=1  SampleTime=1e-08
  ABS : Abs  SampleTime=1e-08  OutDataTypeStr=fixdt(1, 38, 32)  SaturateOnIntegerOverflow=off
  Add1 : Sum  AccumDataTypeStr=fixdt(1, 38, 32)  OutDataTypeStr=fixdt(1, 38, 32)  SampleTime=1e-08
  Add2 : Sum  Inputs=+-  AccumDataTypeStr=fixdt(1, 38, 32)  OutDataTypeStr=fixdt(1, 38, 32)  SampleTime=1e-08
  Add3 : Sum  AccumDataTypeStr=int16  OutDataTypeStr=int16  SampleTime=1e-08
  Constant : Constant  Value=0  OutDataTypeStr=fixdt(1, 38, 32)  SampleTime=1e-08
  Constant1 : Constant  Value=0  OutDataTypeStr=fixdt(1, 38, 32)  SampleTime=1e-08
  Constant2 : Constant  Value=0  OutDataTypeStr=fixdt(1, 38, 32)  SampleTime=1e-08
  Constant3 : Constant  Value=0  OutDataTypeStr=int8  SampleTime=1e-08
  Constant4 : Constant  OutDataTypeStr=int8  SampleTime=1e-08
  Data Type Conversion1 : DataTypeConversion  OutDataTypeStr=boolean  SampleTime=1e-08  SaturateOnIntegerOverflow=off  RndMeth=Floor
  Detec_edge : Sum  Inputs=+-  AccumDataTypeStr=int8  OutDataTypeStr=int8  SampleTime=1e-08
  IfFinalState : RelationalOperator  Operator=>  OutDataTypeStr=boolean  SampleTime=1e-08  InputSameDT=off
  OR : Logic  Operator=OR  AllPortsSameDT=off  OutDataTypeStr=boolean  SampleTime=1e-08
  OR1 : Logic  Operator=OR  AllPortsSameDT=off  OutDataTypeStr=boolean  SampleTime=1e-08
  OnlyAllowInNewPeriod : Switch  Criteria=u2 ~= 0  Threshold=double(0)  OutDataTypeStr=uint16  SampleTime=1e-08  SaturateOnIntegerOverflow=off  InputSameDT=off
  ProtectOverflow_T_count : Switch  Threshold=double(30)  OutDataTypeStr=fixdt(1, 38, 32)  SampleTime=1e-08  SaturateOnIntegerOverflow=off  InputSameDT=off
  ProtectOverflow_rps : Switch  Threshold=double(30)  OutDataTypeStr=fixdt(1, 38, 32)  SampleTime=1e-08  SaturateOnIntegerOverflow=off  InputSameDT=off
  ProtectToUseOmegaIfThetaJump1 : RelationalOperator  Operator=>  OutDataTypeStr=fixdt(1,16,0)  SampleTime=1e-08  InputSameDT=off
  Relational Operator : RelationalOperator  Operator===  OutDataTypeStr=boolean  SampleTime=1e-08  InputSameDT=off
  Reset : Switch  Criteria=u2 ~= 0  Threshold=double(0)  OutDataTypeStr=fixdt(1, 24, 11)  SampleTime=1e-08  SaturateOnIntegerOverflow=off  InputSameDT=off
  Reset1 : Switch  Criteria=u2 ~= 0  Threshold=double(0)  OutDataTypeStr=uint16  SampleTime=1e-08  SaturateOnIntegerOverflow=off  InputSameDT=off
  Reset2 : Switch  Criteria=u2 ~= 0  Threshold=double(0)  OutDataTypeStr=fixdt(1, 24, 11)  SampleTime=1e-08  SaturateOnIntegerOverflow=off  InputSameDT=off
  T_count_switch : Switch  Criteria=u2 > Threshold  Threshold=double(0)  OutDataTypeStr=fixdt(1, 38, 32)  SampleTime=1e-08  SaturateOnIntegerOverflow=off  InputSameDT=off
  adder : Sum  AccumDataTypeStr=uint32  OutDataTypeStr=uint32  SampleTime=1e-08
  const : Constant  Value=0  VectorParams1D=off  OutDataTypeStr=uint32  SampleTime=1e-08
  invt_mult : Subsystem
  omega_registered : Switch  Criteria=u2 ~= 0  Threshold=double(0)  OutDataTypeStr=fixdt(1, 24, 11)  SampleTime=1e-08  SaturateOnIntegerOverflow=off  InputSameDT=off
  rd_{0..10,13} (12 alike) : Delay  DelayLength=double(1)  InitialCondition=0  SampleTime=1e-08
  rd_11 : Delay  DelayLength=double(2)  InitialCondition=0  SampleTime=1e-08
  rd_12 : Delay  DelayLength=double(19)  InitialCondition=0  SampleTime=1e-08
  reset_old_switch1 : Switch  Criteria=u2 ~= 0  Threshold=double(0)  OutDataTypeStr=boolean  SampleTime=1e-08  SaturateOnIntegerOverflow=off  InputSameDT=off
  speed_old_switch : Switch  Criteria=u2 ~= 0  Threshold=double(0)  OutDataTypeStr=fixdt(1, 38, 32)  SampleTime=1e-08  SaturateOnIntegerOverflow=off  InputSameDT=off
  speed_old_switch2 : Switch  Threshold=double(1)  OutDataTypeStr=fixdt(1, 38, 32)  SampleTime=1e-08  SaturateOnIntegerOverflow=off  InputSameDT=off
  step_value : Constant  VectorParams1D=off  OutDataTypeStr=uint32  SampleTime=1e-08
  switchReset : Switch  Criteria=u2 ~= 0  Threshold=double(0)  OutDataTypeStr=uint32  SampleTime=1e-08  SaturateOnIntegerOverflow=off  InputSameDT=off
  t : hdlmdlgenlib/Buffer
  t1 : hdlmdlgenlib/Buffer
  timeout_latch : Switch  Criteria=u2 ~= 0  Threshold=double(0)  OutDataTypeStr=boolean  SampleTime=1e-08  SaturateOnIntegerOverflow=off  InputSameDT=off
  zero_speed_at_timeout : Constant  Value=0  OutDataTypeStr=fixdt(1, 24, 11)  SampleTime=1e-08
  omega_oversampled : Outport  SampleTime=1e-08  VectorParamsAs1DForOutWhenUnconnected=off
  NewMeasurement : Outport  Port=2  SampleTime=1e-08  VectorParamsAs1DForOutWhenUnconnected=off
  state_count_edges : Outport  Port=3  SampleTime=1e-08  VectorParamsAs1DForOutWhenUnconnected=off
  timeout_active : Outport  Port=4  OutDataTypeStr=boolean  SampleTime=1e-08  VectorParamsAs1DForOutWhenUnconnected=off
  wires:
  Encoder Line/1 -> Detec_edge/1, reset_old_switch1/1
  Dir/1 -> speed_old_switch2/2
  T/1 -> Add1/2, Add2/2
  oversampling_state/1 -> OnlyAllowInNewPeriod/1
  timeout_value/1 -> Relational Operator/2
  zero_speed_at_timeout/1 -> Reset2/1
  timeout_latch/1 -> rd_6/1, Reset2/2, timeout_active/1
  speed_old_switch2/1 -> T_count_switch/3, speed_old_switch/1
  omega_registered/1 -> rd_13/1, Reset2/3
  invt_mult/1(omega_oversampled) -> rd_11/1
  Reset2/1 -> omega_oversampled/1
  Reset1/1 -> rd_10/1, invt_mult/3(Oversampling Factor)
  Relational Operator/1 -> rd_2/1, OR/1, timeout_latch/1
  ProtectToUseOmegaIfThetaJump1/1 -> Data Type Conversion1/1, Add3/1
  ProtectOverflow_rps/1 -> invt_mult/2(rps)
  OR/1 -> timeout_latch/2, invt_mult/1(New_Measurement)
  IfFinalState/1 -> OR/2, OnlyAllowInNewPeriod/2, Reset/2, T_count_switch/2, speed_old_switch/2, Reset1/2
  Detec_edge/1 -> rd_1/1, reset_old_switch1/2
  Data Type Conversion1/1 -> OR1/1
  Constant4/1 -> Reset/1
  Constant3/1 -> ProtectToUseOmegaIfThetaJump1/2
  Constant2/1 -> ProtectOverflow_rps/1
  Constant1/1 -> ProtectOverflow_T_count/1
  Constant/1 -> T_count_switch/1
  const/1 -> switchReset/1
  step_value/1 -> adder/2
  adder/1 -> switchReset/3
  OR1/1 -> switchReset/2
  t1/1 -> Relational Operator/1
  Reset/1 -> Add3/2
  Add3/1 -> t/1
  Add2/1 -> speed_old_switch2/3
  ProtectOverflow_T_count/1 -> Add1/1, Add2/1
  Add1/1 -> speed_old_switch2/1
  T_count_switch/1 -> rd_7/1, ABS/1
  rd_2/1 -> OR1/2
  rd_10/1 -> Reset1/3
  rd_7/1 -> ProtectOverflow_T_count/3
  rd_13/1 -> omega_registered/3
  rd_6/1 -> timeout_latch/3
  rd_1/1 -> ProtectToUseOmegaIfThetaJump1/1
  rd_11/1 -> omega_registered/1
  speed_old_switch/1 -> rd_9/1
  rd_9/1 -> speed_old_switch/3, ProtectOverflow_rps/3
  invt_mult/2(New_Measurement_delayed) -> rd_12/1
  rd_12/1 -> NewMeasurement/1, omega_registered/2
  t/1 -> rd_5/1
  rd_5/1 -> Reset/3, state_count_edges/1, IfFinalState/1
  ABS/1 -> rd_8/1
  rd_8/1 -> ProtectOverflow_rps/2, ProtectOverflow_T_count/2
  reset_old_switch1/1 -> rd_0/1
  rd_0/1 -> reset_old_switch1/3, Detec_edge/2
  switchReset/1 -> rd_3/1
  rd_3/1 -> t1/1, adder/1
  OnlyAllowInNewPeriod/1 -> rd_4/1
  rd_4/1 -> OnlyAllowInNewPeriod/3, IfFinalState/2, Reset1/1
